simulink model "model02_quick"  (Simulink 7.9)
settings: Solver=ode45  StartTime=0.0  StopTime=10.0  RelTol=1e-3
undefined symbols (not defined in the file): initE, Kp, T
settings Model: Creator=ex16  LastModifiedBy=ex16

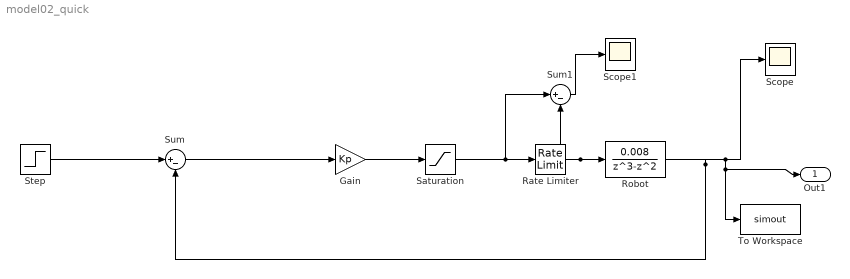
== system model02_quick ==
  Gain : Gain  Gain=Kp  SampleTime=T
  Rate Limiter : RateLimiter  RisingSlewLimit=15  FallingSlewLimit=-15  SampleTimeMode=inherited
  Robot : DiscreteTransferFcn  Numerator=[0.008]  Denominator=[1 -1 0 0]  SampleTime=T
  Saturation : Saturate  UpperLimit=3.2  LowerLimit=-3.2  SampleTime=T
  Scope : Scope
  Scope1 : Scope
  Step : Step  Time=0  After=initE  SampleTime=T
  Sum : Sum  Inputs=|+-
  Sum1 : Sum  Inputs=|+-
  To Workspace : ToWorkspace  VariableName=simout  SampleTime=-1  SaveFormat=Structure With Time
  Out1 : Outport
  wires:
  Gain/1 -> Saturation/1
  Sum/1 -> Gain/1
  Robot/1 -> Sum/2, Scope/1, To Workspace/1, Out1/1
  Saturation/1 -> Rate Limiter/1, Sum1/1
  Rate Limiter/1 -> Robot/1, Sum1/2
  Step/1 -> Sum/1
  Sum1/1 -> Scope1/1
